simulink library "AIV_WetBulbTemperature"  (R2013b)
settings: Solver=ode45  StartTime=0.0  StopTime=10.0  RelTol=1e-3
undefined symbols (not defined in the file): FluidMix, Pressure, Temperature
libraries: carnot x5
settings Model: Creator=lena.frank  LastModifiedBy=drhf

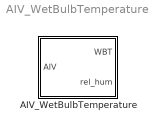
== system AIV_WetBulbTemperature ==
  AIV_WetBulbTemperature : Subsystem  mask(AIV to wet bulb temperature and relative humidity){}
      mask help:
      | Calculate  - the relative humidity of air (rH)
      |                  - and the wet bulb temperature of air (WBT)
      | from          - dry bulb air temperature (DBT)
      |                  - and mass of water per mass of air (x)
      | in AIV vector.
      |
      | DBT        [degree centigrade]
      | p              [Pa]
      | x              kg water / kg air
      |
      | rel_hum   [percent]
      | WBT       [degree centigrade] -> T_WBT is valid for T [-6..40°C]
      mask Help: web(fullfile(path_carnot('help'),'wetbulbtemperature.html'),'-helpbrowser')

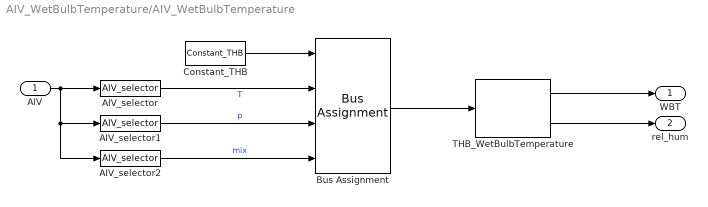
== system AIV_WetBulbTemperature/AIV_WetBulbTemperature ==
  AIV : Inport
  AIV_selector : carnot/Outputs/AIV_selector  e1=off  e2=on  e3=off  e4=off  e5=off  e6=off  e7=off  e8=off  e9=off
  AIV_selector1 : carnot/Outputs/AIV_selector  e1=off  e2=off  e3=off  e4=off  e5=off  e6=off  e7=off  e8=on  e9=off
  AIV_selector2 : carnot/Outputs/AIV_selector  e1=off  e2=off  e3=off  e4=on  e5=off  e6=off  e7=off  e8=off  e9=off
  Bus Assignment : BusAssignment  AssignedSignals=Temperature,Pressure,FluidMix
  Constant_THB : carnot/Source/Simple/Constant_THB  t=20  mdot=0  p=1e5  mID=No Pressure Drop  fluid=Air  mix=0  dia=0.02  hgt=0
  THB_WetBulbTemperature : carnot/Basic/Material_Properties/THB_WetBulbTemperature
  WBT : Outport
  rel_hum : Outport  Port=2
  wires:
  THB_WetBulbTemperature/1 -> WBT/1
  AIV/1 -> AIV_selector1/1, AIV_selector2/1, AIV_selector/1
  AIV_selector/1 -> Bus Assignment/2  "T"
  AIV_selector2/1 -> Bus Assignment/4  "mix"
  AIV_selector1/1 -> Bus Assignment/3  "p"
  Constant_THB/1 -> Bus Assignment/1
  Bus Assignment/1 -> THB_WetBulbTemperature/1
  THB_WetBulbTemperature/2 -> rel_hum/1
